simulink model "ActiveSensing_v2"  (R2019b)
settings: Solver=FixedStepAuto  StartTime=0.0  StopTime=10  FixedStep=0.001  RelTol=1e-3
libraries: simulink x4
settings Model: Creator=BC  LastModifiedBy=boc5244
settings DataIOCC: ReturnWorkspaceOutputs=off
settings DebuggingCC: ArithmeticOperatorsInVariantConditions=warning
settings SFSimCC: SimUseLocalCustomCode=off  CustomCodeUndefinedFunction=UseInterfaceOnly
settings RTWCC: RTWUseLocalCustomCode=off

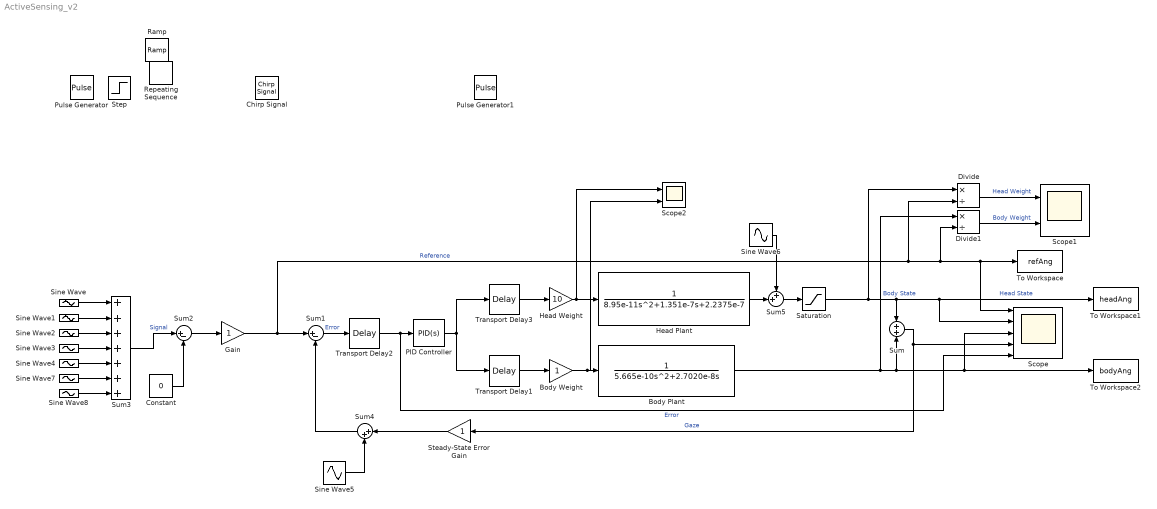
== system ActiveSensing_v2 ==
  Body Weight : Gain
  Body Plant : TransferFcn  Denominator=[5.665e-10 2.7020e-8 0]
  Chirp Signal : simulink/Sources/Chirp Signal  f1=0.1  T=8  f2=12  VectorParams1D=off
  Constant : Constant  Value=0
  Divide : Product  Inputs=*/
  Divide1 : Product  Inputs=*/
  Gain : Gain
  Head Weight : Gain  Gain=10
  Head Plant : TransferFcn  Denominator=[8.95e-11 1.351e-7 2.2375e-7]
  PID Controller : simulink/Continuous/PID Controller  Controller=PID  Form=Parallel  TimeDomain=Continuous-time  SampleTime=-1  IntegratorMethod=Forward Euler  FilterMethod=Forward Euler  ControllerParametersSource=internal  P=4.14023763120658e-07  I=4.0891405375782e-06  D=4.29449375174622e-09  UseFilter=on  N=115.193163393173  TunerSelectOption=Transfer Function Based (PID Tuner App)  InitialConditionSource=internal  InitialConditionForIntegrator=0  InitialConditionForFilter=0  DifferentiatorICPrevScaledInput=0  ExternalReset=none  TrackingMode=off  Kt=1  LimitOutput=off  UpperSaturationLimit=inf  LowerSaturationLimit=-inf  LinearizeAsGain=on  AntiWindupMode=none  Kb=1  POutMin=[]  POutMax=[]  IOutMin=[]  IOutMax=[]  DOutMin=[]  DOutMax=[]  NOutMin=[]  NOutMax=[]  SumOutMin=[]  SumOutMax=[]  SaturationOutMin=[]  SaturationOutMax=[]  PParamMin=[]  PParamMax=[]  IParamMin=[]  IParamMax=[]  DParamMin=[]  DParamMax=[]  NParamMin=[]  NParamMax=[]  KbParamMin=[]  KbParamMax=[]  KtParamMin=[]  KtParamMax=[]  KbOutMin=[]  KbOutMax=[]  KtOutMin=[]  KtOutMax=[]  IntegratorOutMin=[]  IntegratorOutMax=[]  FilterOutMin=[]  FilterOutMax=[]  SumI1OutMin=[]  SumI1OutMax=[]  SumI2OutMin=[]  SumI2OutMax=[]  SumI3OutMin=[]  SumI3OutMax=[]  SumI4OutMin=[]  SumI4OutMax=[]  SumDOutMin=[]  SumDOutMax=[]  DifferentiatorOutMin=[]  DifferentiatorOutMax=[]  FilterDiffOutCoefMin=[]  FilterDiffOutCoefMax=[]  ReciprocalOutMin=[]  ReciprocalOutMax=[]  SumDenOutMin=[]  SumDenOutMax=[]  SumNumOutMin=[]  SumNumOutMax=[]  DivideOutMin=[]  DivideOutMax=[]  IntegratorContinuousStateAttributes=''  IntegratorStateMustResolveToSignalObject=off  IntegratorRTWStateStorageClass=Auto  FilterContinuousStateAttributes=''  FilterStateMustResolveToSignalObject=off  FilterRTWStateStorageClass=Auto  ParallelPVariant=InternalParameters  IdealPVariant=Disabled  IVariant=InternalParameters  DVariant=InternalParameters  IntegratorVariant=Continuous  SatVariant=Disabled  AWVariant=Passthrough  PCopyVariant=Disabled  TRVariant=Disabled  FdbkBlocksVariant=Forward  IdealPFdbkVariant=Disabled  SatFdbkVariant=Disabled  DerivativeFilterVariant=ContFilter  NVariant=InternalParameters  NCopyVariant=Disabled  FilterICVariant=InternalICsFilter  IntegratorICVariant=InternalICs  ExternalResetVariant=Disabled  TRSumVariant=Passthrough  SumFdbkVariant=Disabled  SumVariant=Sum_PID
  Pulse Generator : DiscretePulseGenerator  PulseType=Time based  Period=5  PulseWidth=50
  Pulse Generator1 : DiscretePulseGenerator  PulseType=Time based  Amplitude=20  PulseWidth=50
  Ramp : simulink/Sources/Ramp  slope=30  start=0  InitialOutput=0
  Repeating Sequence : simulink/Sources/Repeating Sequence  rep_seq_t=[0 1 2 3 4 5]  rep_seq_y=[0 30 0 90 0 150]
  Saturation : Saturate  UpperLimit=17  LowerLimit=-17
  Scope : Scope  NumInputPorts=5
  Scope1 : Scope  NumInputPorts=2
  Scope2 : Scope  NumInputPorts=2
  Sine Wave : Sin  Amplitude=10  Frequency=2*pi*0.5  Phase=1.2  SampleTime=0
  Sine Wave1 : Sin  Amplitude=10  Frequency=2*pi*1.4  Phase=0.77  SampleTime=0
  Sine Wave2 : Sin  Amplitude=10  Frequency=2*pi*3.3  Phase=2.4  SampleTime=0
  Sine Wave3 : Sin  Amplitude=10  Frequency=2*pi*7.6  Phase=0.664565  SampleTime=0
  Sine Wave4 : Sin  Amplitude=10  Frequency=2*pi*10  Phase=0.1786  SampleTime=0
  Sine Wave5 : Sin  Amplitude=0  Frequency=20  SampleTime=0
  Sine Wave6 : Sin  Amplitude=0  Frequency=16  SampleTime=0
  Sine Wave7 : Sin  Amplitude=0  Frequency=2*pi*0.2  Phase=0.8925  SampleTime=0
  Sine Wave8 : Sin  Amplitude=0  Frequency=2*pi*20  Phase=0.1786  SampleTime=0
  Steady-State Error Gain : Gain
  Step : Step  Time=0.1  After=50  SampleTime=0
  Sum : Sum  Inputs=+|+
  Sum1 : Sum  Inputs=|+-
  Sum2 : Sum  Inputs=|+-
  Sum3 : Sum  Inputs=+++++++
  Sum4 : Sum  Inputs=|++
  Sum5 : Sum  Inputs=++|
  To Workspace : ToWorkspace  VariableName=refAng  SampleTime=-1
      settings: Save2DSignal=2-D array (concatenate along first dimension)
  To Workspace1 : ToWorkspace  VariableName=headAng  SampleTime=-1
      settings: Save2DSignal=2-D array (concatenate along first dimension)
  To Workspace2 : ToWorkspace  VariableName=bodyAng  SampleTime=-1
      settings: Save2DSignal=2-D array (concatenate along first dimension)
  Transport Delay1 : TransportDelay  DelayTime=0
  Transport Delay2 : TransportDelay  DelayTime=0
  Transport Delay3 : TransportDelay  DelayTime=0
  wires:
  Body Plant/1 -> Divide1/1, Sum/2, To Workspace2/1, Scope/3  "Body State"
  Sum1/1 -> Transport Delay2/1  "Error"
  Head Weight/1 -> Head Plant/1, Scope2/1
  Body Weight/1 -> Scope2/2, Body Plant/1
  PID Controller/1 -> Transport Delay3/1, Transport Delay1/1
  Sum/1 -> Steady-State Error Gain/1, Scope/4  "Gaze"
  Saturation/1 -> Divide/1, To Workspace1/1, Scope/2, Sum/1  "Head State"
  Gain/1 -> Divide/2, Divide1/2, Scope/1, To Workspace/1, Sum1/1  "Reference"
  Transport Delay3/1 -> Head Weight/1
  Transport Delay1/1 -> Body Weight/1
  Transport Delay2/1 -> PID Controller/1, Scope/5  "Error"
  Sum2/1 -> Gain/1
  Constant/1 -> Sum2/2
  Divide/1 -> Scope1/1  "Head Weight"
  Divide1/1 -> Scope1/2  "Body Weight"
  Sum4/1 -> Sum1/2
  Sine Wave5/1 -> Sum4/2
  Head Plant/1 -> Sum5/2
  Sum5/1 -> Saturation/1
  Sine Wave6/1 -> Sum5/1
  Steady-State Error Gain/1 -> Sum4/1
  Sine Wave4/1 -> Sum3/5
  Sine Wave/1 -> Sum3/1
  Sine Wave2/1 -> Sum3/3
  Sine Wave3/1 -> Sum3/4
  Sum3/1 -> Sum2/1  "Signal"
  Sine Wave1/1 -> Sum3/2
  Sine Wave7/1 -> Sum3/6
  Sine Wave8/1 -> Sum3/7
